simulink model "sensors"  (R2024a)
settings: configuration reference "standardSILConfiguraitonParams" (kept outside this file)
settings Model: Creator=GTAR  LastModifiedBy=jerem
settings ConfigSetRef: SourceName=standardSILConfiguraitonParams  SourceLocation=Base Workspace

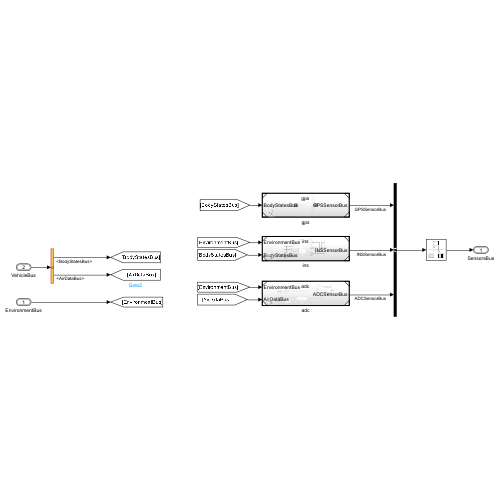
[thumbnail: Simulink's stored preview of the top-level diagram]
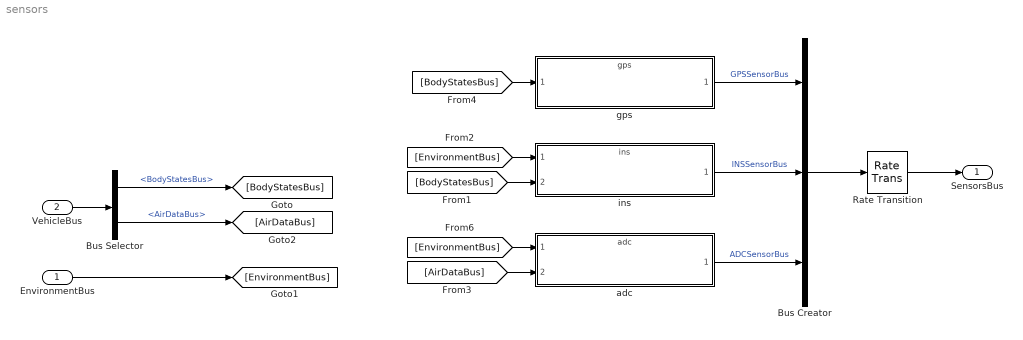
== system sensors ==
  EnvironmentBus : Inport  OutDataTypeStr=Bus: EnvironmentBus
  VehicleBus : Inport  Port=2  OutDataTypeStr=Bus: VehicleBus
  Bus Creator : BusCreator  Inputs=3  OutDataTypeStr=Bus: SensorsBus
      settings: InheritFromInputs=off
  Bus Selector : BusSelector  OutputSignals=BodyStatesBus,AirDataBus
  Rate Transition : RateTransition
  adc : ModelReference  ModelNameDialog=adc.slx  SimulationMode=Normal  ModelReferenceVersion=1.68
  gps : ModelReference  ModelNameDialog=gps.slx  SimulationMode=Normal  ModelReferenceVersion=1.43
  ins : ModelReference  ModelNameDialog=ins.slx  SimulationMode=Normal  ModelReferenceVersion=1.45
  SensorsBus : Outport  OutDataTypeStr=Bus: SensorsBus  BusOutputAsStruct=on
  wires:
  Bus Creator/1 -> Rate Transition/1
  VehicleBus/1 -> Bus Selector/1
  Bus Selector/1 -> [BodyStatesBus]  "<BodyStatesBus>"
  EnvironmentBus/1 -> [EnvironmentBus]
  [EnvironmentBus] -> ins/1
  [BodyStatesBus] -> ins/2
  [AirDataBus] -> adc/2
  [EnvironmentBus] -> adc/1
  ins/1 -> Bus Creator/2  "INSSensorBus"
  [BodyStatesBus] -> gps/1
  Bus Selector/2 -> [AirDataBus]  "<AirDataBus>"
  Rate Transition/1 -> SensorsBus/1
  gps/1 -> Bus Creator/1  "GPSSensorBus"
  adc/1 -> Bus Creator/3  "ADCSensorBus"
